simulink model "scenario1_TAC_5robots_plus_2019"  (R2019a)
settings: Solver=FixedStepAuto  StartTime=0.0  StopTime=40.0  FixedStep=1e-2  RelTol=1e-3
libraries: simulink x6
(part 2 of 2)

== matlab function scenario1_TAC_5robots_plus_2019/distance ==
  data: agent1_x1 input; distance_1_2 output; agent1_x2 input; agent2_x1 input; agent2_x2 input; agent3_x1 input; agent3_x2 input; agent4_x1 input; agent4_x2 input; agent5_x1 input; agent5_x2 input; distance_1_3 output; distance_1_4 output; distance_1_5 output; distance_2_3 output; distance_2_4 output; distance_2_5 output; distance_3_4 output; distance_3_5 output; distance_4_5 output
function [distance_1_2,distance_1_3,distance_1_4,distance_1_5,distance_2_3,distance_2_4,distance_2_5,distance_3_4,distance_3_5,distance_4_5]  = fcn(agent1_x1,agent1_x2,agent2_x1,agent2_x2,agent3_x1,agent3_x2,agent4_x1,agent4_x2,agent5_x1,agent5_x2)
distance_1_2=sqrt( (agent1_x1-agent2_x1)^2+ (agent1_x2-agent2_x2 )^2  );
distance_1_3=sqrt( (agent1_x1-agent3_x1)^2+ (agent1_x2-agent3_x2 )^2  );
distance_1_4=sqrt( (agent1_x1-agent4_x1)^2+ (agent1_x2-agent4_x2 )^2  );
distance_1_5=sqrt( (agent1_x1-agent5_x1)^2+ (agent1_x2-agent5_x2 )^2  );
distance_2_3=sqrt( (agent2_x1-agent3_x1)^2+ (agent2_x2-agent3_x2 )^2  );
distance_2_4=sqrt( (agent2_x1-agent4_x1)^2+ (agent2_x2-agent4_x2 )^2  );
distance_2_5=sqrt( (agent2_x1-agent5_x1)^2+ (agent2_x2-agent5_x2 )^2  );
distance_3_4=sqrt( (agent3_x1-agent4_x1)^2+ (agent3_x2-agent4_x2 )^2  );
distance_3_5=sqrt( (agent3_x1-agent5_x1)^2+ (agent3_x2-agent5_x2 )^2  );
distance_4_5=sqrt( (agent4_x1-agent5_x1)^2+ (agent4_x2-agent5_x2 )^2  );

== matlab function scenario1_TAC_5robots_plus_2019/agent_3/MATLAB Function ==
  data: x1 input; theta output; y1 input
function theta = fcn(x1, y1)
theta=atan2(y1,x1);

== matlab function scenario1_TAC_5robots_plus_2019/agent_3/MATLAB Function1 ==
  data: STL_u1 input; U1 output; STL_u2 input; STL_u3 input; PFM_u1 input; PFM_u2 input; PFM_u3 input; b1 input; U2 output; U3 output
function [U1,U2,U3] = fcn(STL_u1,STL_u2,STL_u3,PFM_u1,PFM_u2,PFM_u3,b1)
U_goal=[STL_u1;STL_u2;STL_u3];
U_obs=[PFM_u1;PFM_u2;PFM_u3];
k=0.15;
lambda=1-exp(-k*max(b1,0));
U=lambda*U_goal+(1-lambda)*U_obs;
U1=0;U2=0;U3=0;
U1=U(1,1);
U2=U(2,1);
U3=U(3,1);

== matlab function scenario1_TAC_5robots_plus_2019/agent_3/MATLAB Function2 ==
  data: v1 input; v output; v2 input
function v = fcn(v1, v2)
v=sqrt(v1^2+v2^2);

== matlab function scenario1_TAC_5robots_plus_2019/agent_3/Potential_Field_controller ==
  data: x1 input; x2 input; u1 output; xa3 input; agent1_x1 input; agent1_x2 input; agent2_x1 input; agent2_x2 input; agent4_x1 input; agent4_x2 input; agent5_x1 input; agent5_x2 input; t input; u2 output; u3 output; v_max input; yita output
function [u1,u2,u3,yita] = fcn(x1, x2, xa3,agent1_x1,agent1_x2,agent2_x1,agent2_x2,agent4_x1,agent4_x2,agent5_x1,agent5_x2,t,v_max)
coder.extrinsic('Calculate_gradient');
coder.extrinsic('Calculate_gradient_V1');
coder.extrinsic('Calculate_gradient_V1_yita');
coder.extrinsic('Calculate_gradient_static_d_1');
coder.extrinsic('Calculate_gradient_static_d_2');
coder.extrinsic('Calculate_gradient_dynamic');
coder.extrinsic('compute_convex_hull');
coder.extrinsic('PVF_optimizer');
coder.extrinsic('add_random');
yita=0;

A1=[-1,0;0,-1];
if t<20
    F=[100,0];
elseif t>=20 && t<41
     F=[200,200];
else
    F=[200,0];
end
obs=[50,50];
Robs_s=20;
r_obs=16;
distance=sqrt((x1-90)^2+(x2-90)^2);
gradient_x=0;gradient_y=0;
Dgradient_x=0;Dgradient_y=0;
agent1_gradient_x=0;agent1_gradient_y=0;
agent2_gradient_x=0;agent2_gradient_y=0;
agent4_gradient_x=0;agent4_gradient_y=0;
agent5_gradient_x=0;agent5_gradient_y=0;
[gradient_x,gradient_y]=Calculate_gradient(x1,x2,A1,F,50,50,Robs_s);
[agent1_gradient_x,agent1_gradient_y]=Calculate_gradient_dynamic(x1,x2,A1,F,agent1_x1,agent1_x2,10);
[agent2_gradient_x,agent2_gradient_y]=Calculate_gradient_dynamic(x1,x2,A1,F,agent2_x1,agent2_x2,10);
[agent4_gradient_x,agent4_gradient_y]=Calculate_gradient_dynamic(x1,x2,A1,F,agent4_x1,agent4_x2,10);
[agent5_gradient_x,agent5_gradient_y]=Calculate_gradient_dynamic(x1,x2,A1,F,agent5_x1,agent5_x2,10);
if sqrt((x1-agent1_x1)^2+(x2-agent1_x2)^2)<=30 %agent3 and agent1
     gradient_x=gradient_x+agent1_gradient_x;
     gradient_y=gradient_y+agent1_gradient_y;
end
if sqrt((x1-agent2_x1)^2+(x2-agent2_x2)^2)<=30 %agent3 and agent2
     gradient_x=gradient_x+agent2_gradient_x;
     gradient_y=gradient_y+agent2_gradient_y;
end
if sqrt((x1-agent4_x1)^2+(x2-agent4_x2)^2)<=30 %agent3 and agent4
     gradient_x=gradient_x+agent4_gradient_x;
     gradient_y=gradient_y+agent4_gradient_y;
end
if sqrt((x1-agent5_x1)^2+(x2-agent5_x2)^2)<=30 %agent3 and agent5
     gradient_x=gradient_x+agent5_gradient_x;
     gradient_y=gradient_y+agent5_gradient_y;
end
gradient_x=gradient_x;
gradient_y=gradient_y;  
gradient_z=0;
Gradient_all=[gradient_x;gradient_y;gradient_z];



Li=0.2;
Bi=[0,cos(pi/6),-cos(pi/6);
    -1,sin(pi/6),sin(pi/6);
    Li,Li,Li;];

R1=[cos(xa3),-sin(xa3),0;
    sin(xa3),cos(xa3),0;
    0,0,1;];
R=0.02;

gx=R1*inv(Bi')*R;
A=Gradient_all'*gx;
% A=[A;-gx];
%H=[1];
%H=[1,0;0,1];
%H=[0,0,0;0,0,0;0,0,0];

 H1=[1,0,0;0,1,0;0,0,0];
 H=(1/2)*gx'*H1*gx;
b=[0];
% b=[0;5000;5000;5000];
Gain=50;
Gradient_final=Gain*Gradient_all;
F=[-2*gx'*H1'*Gradient_final];
%=[];
u1=0;u2=0;u3=0;
U=PVF_optimizer(H,b,A,F,distance,gradient_x,gradient_y);

u1=U(1,1);
u2=U(2,1);
u3=U(3,1);

== matlab function scenario1_TAC_5robots_plus_2019/agent_3/STL_barrier  ==
  data: b output; b1 output; yita output; h output; t input; p1 input; p2 input; agent1_x1 input; agent1_x2 input; agent2_x1 input; agent2_x2 input; agent4_x1 input; agent4_x2 input; agent5_x1 input; agent5_x2 input
function [b,b1,yita,h] = fcn(t,p1,p2,agent1_x1,agent1_x2,agent2_x1,agent2_x2,agent4_x1,agent4_x2,agent5_x1,agent5_x2)
if t<20
    d1=50;
    d2=0;
elseif t>=20 && t<41
    d1=100;
    d2=100;
else
    d1=100;
    d2=0;  
end

obs1=50;
obs2=50;
if t<20
b=105*exp(-0.22*t)+5-sqrt( (p1-d1)^2 + (p2-d2)^2 );
yita=-105*exp(-0.22*t)+5;
h=10-sqrt( (p1-d1)^2 + (p2-d2)^2 );
elseif t>=20 && t<41
    b=110*exp(-0.22*(t-20))+5-sqrt( (p1-d1)^2 + (p2-d2)^2 );
   yita=-110*exp(-0.22*(t-20))+5;
    h=10-sqrt( (p1-d1)^2 + (p2-d2)^2 );
else
   b=145*exp(-0.24*(t-40))+5-sqrt( (p1-d1)^2 + (p2-d2)^2 );
   yita=-145*exp(-0.24*(t-40))+5;
   h=10-sqrt( (p1-d1)^2 + (p2-d2)^2 );
end
% b11=sqrt( (p1-x1_agent2)^2 + (p2-x2_agent2)^2 )-10 %collision avoidence with agent2
bobs=sqrt( (p1-obs1)^2 + (p2-obs2)^2 )-20;%collision avoidence with obstacle (50,50)
b31=sqrt( (p1-agent1_x1)^2 + (p2-agent1_x2)^2 )-10;%collision avoidence with agent1
b32=sqrt( (p1-agent2_x1)^2 + (p2-agent2_x2)^2 )-10;%collision avoidence with agent2
b34=sqrt( (p1-agent4_x1)^2 + (p2-agent4_x2)^2 )-10;%collision avoidence with agent4
b35=sqrt( (p1-agent5_x1)^2 + (p2-agent5_x2)^2 )-10;%collision avoidence with agent5
% b13=sqrt( (p1-centerjk_1)^2 + (p2-centerjk_2)^2 )-R_jk_s;%collision avoidence with nominal
% b14=sqrt( (p1-60)^2 + (p2-85)^2 )-18; %static dynamic obstacle
% b15=sqrt( (p1-20)^2 + (p2-80)^2 )-10; %static dynamic obstacle


b1=-(1/20)*log(exp(-20*bobs)+exp(-20*b31)+exp(-20*b32)+exp(-20*b34)+exp(-20*b35));

% b1=-(1/20)*log(exp(-20*b11)+exp(-20*b12)+exp(-20*b14)+exp(-20*b15));%+log(2);

== matlab function scenario1_TAC_5robots_plus_2019/agent_3/STL_controller ==
  data: x1 input; x2 input; b_in input; u1 output; xa3 input; u2 output; u3 output; t input; v_max input
function [u1,u2,u3]= fcn(x1, x2, b_in, xa3,t, v_max)
coder.extrinsic('quadoptimizer');
%coder.extrinsic('save');
if t<20
    d1=50; d2=0;
elseif t>=20 && t<41
   d1=100; d2=100; 
else
   d1=100; d2=0; 
end

partial_b=(1/2)*((x1-d1)^2+(x2-d2)^2)^(-1/2);
partial_b_x=[-2*partial_b*(x1-d1),-2*partial_b*(x2-d2),0];


Li=0.2;
Bi=[0,cos(pi/6),-cos(pi/6);
    -1,sin(pi/6),sin(pi/6);
    Li,Li,Li;];

R1=[cos(xa3),-sin(xa3),0;
    sin(xa3),cos(xa3),0;
    0,0,1;];
R=0.02;
gx=R1*inv(Bi')*R;

A=partial_b_x*gx;
% A=[A;-gx];
H=[1,0,0;0,1,0;0,0,1];
%H=[1];
if t<20
    b=5*b_in-0.22*105*exp(-0.22*t)-20;
elseif t>=20 && t<41
    b=5*b_in-0.22*110*exp(-0.22*(t-20))-20;
else
    b=20*b_in-0.24*145*exp(-0.24*(t-40))-100;
end
% b=[b;5000;5000;5000];


u1=0;u2=0;u3=0;
U=[0;0;0];
U=quadoptimizer(H,b,A);

%U=quadprod(H,[],-A,b);
% V=[0;0;0];
% V=gx*U;
% if V(1,1)^2+V(2,1)^2<=v_max^2
%      U(1,1)= U(1,1);
%      U(2,1)= U(2,1);
% else 
%     U(1,1)=sqrt(v_max^2/(V(1,1)^2+V(2,1)^2))*U(1,1);
%     U(2,1)=sqrt(v_max^2/(V(1,1)^2+V(2,1)^2))*U(2,1);
% end


u1=U(1,1);
u2=U(2,1);
u3=U(3,1);

== matlab function scenario1_TAC_5robots_plus_2019/agent_3/omnidirectional robot_1 ==
  data: ua1 input; xa1_dot output; ua2 input; ua3 input; xa3 input; xa2_dot output; xa3_dot output
function [xa1_dot,xa2_dot,xa3_dot]= fcn(ua1,ua2,ua3,xa3)

Li=0.2;
Bi=[0,cos(pi/6),-cos(pi/6);
    -1,sin(pi/6),sin(pi/6);
    Li,Li,Li;];

R1=[cos(xa3),-sin(xa3),0;
    sin(xa3),cos(xa3),0;
    0,0,1;];
R=0.02;
A=R1*inv(Bi')*R*[ua1;ua2;ua3];
xa1_dot=A(1,1);
xa2_dot=A(2,1);
xa3_dot=A(3,1);

== matlab function scenario1_TAC_5robots_plus_2019/agent_3/velocity_constraint ==
  data: U1 input; Uc1 output; U2 input; U3 input; Uc2 output; Uc3 output; xa3 input; v_max input
function [Uc1,Uc2,Uc3] = fcn(U1,U2,U3,xa3,v_max)

Li=0.2;
Bi=[0,cos(pi/6),-cos(pi/6);
    -1,sin(pi/6),sin(pi/6);
    Li,Li,Li;];

R1=[cos(xa3),-sin(xa3),0;
    sin(xa3),cos(xa3),0;
    0,0,1;];
R=0.02;
gx=R1*inv(Bi')*R;

U=[U1;U2;U3];
V=[0;0;0];
V=gx*U;
if V(1,1)^2+V(2,1)^2<=v_max^2
     U(1,1)= U(1,1);
     U(2,1)= U(2,1);
else 
    U(1,1)=sqrt(v_max^2/(V(1,1)^2+V(2,1)^2))*U(1,1);
    U(2,1)=sqrt(v_max^2/(V(1,1)^2+V(2,1)^2))*U(2,1);
    U(3,1)=sqrt(v_max^2/(V(1,1)^2+V(2,1)^2))*U(3,1);
end

Uc1=U(1,1);
Uc2=U(2,1);
Uc3=U(3,1);

== matlab function scenario1_TAC_5robots_plus_2019/agent_4/MATLAB Function ==
  data: x1 input; theta output; y1 input
function theta = fcn(x1, y1)
theta=atan2(y1,x1);

== matlab function scenario1_TAC_5robots_plus_2019/agent_4/MATLAB Function1 ==
  data: STL_u1 input; U1 output; STL_u2 input; STL_u3 input; PFM_u1 input; PFM_u2 input; PFM_u3 input; b1 input; U2 output; U3 output; t input
function [U1,U2,U3] = fcn(STL_u1,STL_u2,STL_u3,PFM_u1,PFM_u2,PFM_u3,b1,t)
U_goal=[STL_u1;STL_u2;STL_u3];
U_obs=[PFM_u1;PFM_u2;PFM_u3];
k=0.15;
lambda=1-exp(-k*max(b1,0));
U=lambda*U_goal+(1-lambda)*U_obs;
U1=0;U2=0;U3=0;
if t<=20
U1=0;
U2=0;
U3=0;    
% U1=U(1,1);
% U2=U(2,1);
% U3=U(3,1);
else
U1=U(1,1);
U2=U(2,1);
U3=U(3,1);
end

== matlab function scenario1_TAC_5robots_plus_2019/agent_4/MATLAB Function2 ==
  data: v1 input; v output; v2 input
function v = fcn(v1, v2)
v=sqrt(v1^2+v2^2);

== matlab function scenario1_TAC_5robots_plus_2019/agent_4/Potential_Field_controller ==
  data: x1 input; x2 input; u1 output; xa3 input; agent1_x1 input; agent1_x2 input; agent2_x1 input; agent2_x2 input; agent3_x1 input; agent3_x2 input; agent5_x1 input; agent5_x2 input; t input; u2 output; u3 output; v_max input; yita output
function [u1,u2,u3,yita] = fcn(x1, x2, xa3,agent1_x1,agent1_x2,agent2_x1,agent2_x2,agent3_x1,agent3_x2,agent5_x1,agent5_x2,t,v_max)
coder.extrinsic('Calculate_gradient');
coder.extrinsic('Calculate_gradient_V1');
coder.extrinsic('Calculate_gradient_V1_yita');
coder.extrinsic('Calculate_gradient_static_d_1');
coder.extrinsic('Calculate_gradient_static_d_2');
coder.extrinsic('Calculate_gradient_dynamic');
coder.extrinsic('compute_convex_hull');
coder.extrinsic('PVF_optimizer');
coder.extrinsic('add_random');
yita=0;

A1=[-1,0;0,-1];
if t<20
    F=[2*(-45*cos(t)+50),2*(45*sin(t)+50)];
elseif t>=20 && t<41
%      F=[0,200];
    F=[2*(-45*cos(t-20)+50),2*(45*sin(t-20)+50)];
else
    F=[200,0];
end
obs=[50,50];
Robs_s=20;
r_obs=16;
distance=sqrt((x1-90)^2+(x2-90)^2);
gradient_x=0;gradient_y=0;
Dgradient_x=0;Dgradient_y=0;
agent1_gradient_x=0;agent1_gradient_y=0;
agent2_gradient_x=0;agent2_gradient_y=0;
agent3_gradient_x=0;agent3_gradient_y=0;
agent5_gradient_x=0;agent5_gradient_y=0;
[gradient_x,gradient_y]=Calculate_gradient(x1,x2,A1,F,50,50,Robs_s);
[agent1_gradient_x,agent1_gradient_y]=Calculate_gradient_dynamic(x1,x2,A1,F,agent1_x1,agent1_x2,10);
[agent2_gradient_x,agent2_gradient_y]=Calculate_gradient_dynamic(x1,x2,A1,F,agent2_x1,agent2_x2,10);
[agent3_gradient_x,agent3_gradient_y]=Calculate_gradient_dynamic(x1,x2,A1,F,agent3_x1,agent3_x2,10);
[agent5_gradient_x,agent5_gradient_y]=Calculate_gradient_dynamic(x1,x2,A1,F,agent5_x1,agent5_x2,10);
if sqrt((x1-agent1_x1)^2+(x2-agent1_x2)^2)<=30 %agent4 and agent1
     gradient_x=gradient_x+agent1_gradient_x;
     gradient_y=gradient_y+agent1_gradient_y;
end
if sqrt((x1-agent2_x1)^2+(x2-agent2_x2)^2)<=30 %agent4 and agent2
     gradient_x=gradient_x+agent2_gradient_x;
     gradient_y=gradient_y+agent2_gradient_y;
end
if sqrt((x1-agent3_x1)^2+(x2-agent3_x2)^2)<=30 %agent4 and agent3
     gradient_x=gradient_x+agent3_gradient_x;
     gradient_y=gradient_y+agent3_gradient_y;
end
if sqrt((x1-agent5_x1)^2+(x2-agent5_x2)^2)<=30 %agent4 and agent5
     gradient_x=gradient_x+agent5_gradient_x;
     gradient_y=gradient_y+agent5_gradient_y;
end
gradient_x=gradient_x;
gradient_y=gradient_y;  
gradient_z=0;
Gradient_all=[gradient_x;gradient_y;gradient_z];



Li=0.2;
Bi=[0,cos(pi/6),-cos(pi/6);
    -1,sin(pi/6),sin(pi/6);
    Li,Li,Li;];

R1=[cos(xa3),-sin(xa3),0;
    sin(xa3),cos(xa3),0;
    0,0,1;];
R=0.02;

gx=R1*inv(Bi')*R;
A=Gradient_all'*gx;
% A=[A;-gx];
%H=[1];
%H=[1,0;0,1];
%H=[0,0,0;0,0,0;0,0,0];

 H1=[1,0,0;0,1,0;0,0,0];
 H=(1/2)*gx'*H1*gx;
b=[0];
% b=[0;5000;5000;5000];
Gain=50;
Gradient_final=Gain*Gradient_all;
F=[-2*gx'*H1'*Gradient_final];
%=[];
u1=0;u2=0;u3=0;
U=PVF_optimizer(H,b,A,F,distance,gradient_x,gradient_y);

u1=U(1,1);
u2=U(2,1);
u3=U(3,1);

== matlab function scenario1_TAC_5robots_plus_2019/agent_4/STL_barrier  ==
  data: b output; b1 output; yita output; h output; t input; p1 input; p2 input; agent1_x1 input; agent1_x2 input; agent2_x1 input; agent2_x2 input; agent3_x1 input; agent3_x2 input; agent5_x1 input; agent5_x2 input
function [b,b1,yita,h] = fcn(t,p1,p2,agent1_x1,agent1_x2,agent2_x1,agent2_x2,agent3_x1,agent3_x2,agent5_x1,agent5_x2)
if t<20
    d1=-45*cos(t)+50;
    d2= 45*sin(t)+50;
elseif t>=20 && t<41
    d1=-45*cos(t-20)+50;
    d2= 45*sin(t-20)+50;
else
    d1=100;
    d2=0;  
end

obs1=50;
obs2=50;
if t<20
% b=105*exp(-0.22*t)+5-sqrt( (p1-d1)^2 + (p2-d2)^2 );
% yita=-105*exp(-0.22*t)+5;
% h=10-sqrt( (p1-d1)^2 + (p2-d2)^2 );
b=7-sqrt( (p1-d1)^2 + (p2-d2)^2 );
yita=3;
h=10-sqrt( (p1-d1)^2 + (p2-d2)^2 );
elseif t>=20 && t<41
%     b=90*exp(-0.208*(t-20))+5-sqrt( (p1-d1)^2 + (p2-d2)^2 );
%    yita=-90*exp(-0.2295*(t-20))+5;
%     h=10-sqrt( (p1-d1)^2 + (p2-d2)^2 );
b=7-sqrt( (p1-d1)^2 + (p2-d2)^2 );
yita=3;
h=10-sqrt( (p1-d1)^2 + (p2-d2)^2 );
else
   b=145*exp(-0.24*(t-40))+5-sqrt( (p1-d1)^2 + (p2-d2)^2 );
   yita=-145*exp(-0.24*(t-40))+5;
   h=10-sqrt( (p1-d1)^2 + (p2-d2)^2 );
end
bobs=sqrt( (p1-obs1)^2 + (p2-obs2)^2 )-20;%collision avoidence with obstacle (50,50)
b41=sqrt( (p1-agent1_x1)^2 + (p2-agent1_x2)^2 )-10;%collision avoidence with agent1
b42=sqrt( (p1-agent2_x1)^2 + (p2-agent2_x2)^2 )-10;%collision avoidence with agent2
b43=sqrt( (p1-agent3_x1)^2 + (p2-agent3_x2)^2 )-10;%collision avoidence with agent3
b45=sqrt( (p1-agent5_x1)^2 + (p2-agent5_x2)^2 )-10;%collision avoidence with agent5

b1=-(1/20)*log(exp(-20*bobs)+exp(-20*b41)+exp(-20*b42)+exp(-20*b43)+exp(-20*b45));

% b1=-(1/20)*log(exp(-20*b11)+exp(-20*b12)+exp(-20*b14)+exp(-20*b15));%+log(2);

== matlab function scenario1_TAC_5robots_plus_2019/agent_4/STL_controller ==
  data: x1 input; x2 input; b_in input; u1 output; xa3 input; u2 output; u3 output; t input; v_max input
function [u1,u2,u3]= fcn(x1, x2, b_in, xa3,t, v_max)
coder.extrinsic('quadoptimizer');
%coder.extrinsic('save');
if t<20
    d1=-45*cos(t)+50; d2=45*sin(t)+50;
elseif t>=20 && t<41
%    d1=0; d2=100; 
    d1=-45*cos(t-20)+50; d2=45*sin(t-20)+50;
else
   d1=100; d2=0; 
end

partial_b=(1/2)*((x1-d1)^2+(x2-d2)^2)^(-1/2);
partial_b_x=[-2*partial_b*(x1-d1),-2*partial_b*(x2-d2),0];
partial_b_t= -2*partial_b*(x1-d1)*(-45*sin(t-20))-2*partial_b*(x2-d2)*(-45*cos(t-20));

Li=0.2;
Bi=[0,cos(pi/6),-cos(pi/6);
    -1,sin(pi/6),sin(pi/6);
    Li,Li,Li;];

R1=[cos(xa3),-sin(xa3),0;
    sin(xa3),cos(xa3),0;
    0,0,1;];
R=0.02;
gx=R1*inv(Bi')*R;

A=partial_b_x*gx;
% A=[A;-gx];
H=[1,0,0;0,1,0;0,0,1];
%H=[1];
if t<20
%     b=5*b_in-0.22*105*exp(-0.22*t)-20;
     b=5*b_in+partial_b_t-10;
elseif t>=20 && t<41
%     b=20*b_in-0.208*90*exp(-0.208*(t-20))-100;
     b=50*b_in+partial_b_t-50;
else
    b=20*b_in-0.24*145*exp(-0.24*(t-40))-100;
end
% b=[b;5000;5000;5000];


u1=0;u2=0;u3=0;
U=[0;0;0];
U=quadoptimizer(H,b,A);

%U=quadprod(H,[],-A,b);
% V=[0;0;0];
% V=gx*U;
% if V(1,1)^2+V(2,1)^2<=v_max^2
%      U(1,1)= U(1,1);
%      U(2,1)= U(2,1);
% else 
%     U(1,1)=sqrt(v_max^2/(V(1,1)^2+V(2,1)^2))*U(1,1);
%     U(2,1)=sqrt(v_max^2/(V(1,1)^2+V(2,1)^2))*U(2,1);
% end


u1=U(1,1);
u2=U(2,1);
u3=U(3,1);

== matlab function scenario1_TAC_5robots_plus_2019/agent_4/omnidirectional robot_1 ==
  data: ua1 input; xa1_dot output; ua2 input; ua3 input; xa3 input; xa2_dot output; xa3_dot output
function [xa1_dot,xa2_dot,xa3_dot]= fcn(ua1,ua2,ua3,xa3)

Li=0.2;
Bi=[0,cos(pi/6),-cos(pi/6);
    -1,sin(pi/6),sin(pi/6);
    Li,Li,Li;];

R1=[cos(xa3),-sin(xa3),0;
    sin(xa3),cos(xa3),0;
    0,0,1;];
R=0.02;
A=R1*inv(Bi')*R*[ua1;ua2;ua3];
xa1_dot=A(1,1);
xa2_dot=A(2,1);
xa3_dot=A(3,1);

== matlab function scenario1_TAC_5robots_plus_2019/agent_4/velocity_constraint ==
  data: U1 input; Uc1 output; U2 input; U3 input; Uc2 output; Uc3 output; xa3 input; v_max input
function [Uc1,Uc2,Uc3] = fcn(U1,U2,U3,xa3,v_max)

Li=0.2;
Bi=[0,cos(pi/6),-cos(pi/6);
    -1,sin(pi/6),sin(pi/6);
    Li,Li,Li;];

R1=[cos(xa3),-sin(xa3),0;
    sin(xa3),cos(xa3),0;
    0,0,1;];
R=0.02;
gx=R1*inv(Bi')*R;

U=[U1;U2;U3];
V=[0;0;0];
V=gx*U;
if V(1,1)^2+V(2,1)^2<=v_max^2
     U(1,1)= U(1,1);
     U(2,1)= U(2,1);
else 
    U(1,1)=sqrt(v_max^2/(V(1,1)^2+V(2,1)^2))*U(1,1);
    U(2,1)=sqrt(v_max^2/(V(1,1)^2+V(2,1)^2))*U(2,1);
    U(3,1)=sqrt(v_max^2/(V(1,1)^2+V(2,1)^2))*U(3,1);
end

Uc1=U(1,1);
Uc2=U(2,1);
Uc3=U(3,1);

== matlab function scenario1_TAC_5robots_plus_2019/agent_5/MATLAB Function ==
  data: x1 input; theta output; y1 input
function theta = fcn(x1, y1)
theta=atan2(y1,x1);

== matlab function scenario1_TAC_5robots_plus_2019/agent_5/MATLAB Function1 ==
  data: STL_u1 input; U1 output; STL_u2 input; STL_u3 input; PFM_u1 input; PFM_u2 input; PFM_u3 input; b1 input; U2 output; U3 output
function [U1,U2,U3] = fcn(STL_u1,STL_u2,STL_u3,PFM_u1,PFM_u2,PFM_u3,b1)
U_goal=[STL_u1;STL_u2;STL_u3];
U_obs=[PFM_u1;PFM_u2;PFM_u3];
k=0.15;
lambda=1-exp(-k*max(b1,0));
U=lambda*U_goal+(1-lambda)*U_obs;
U1=0;U2=0;U3=0;
U1=U(1,1);
U2=U(2,1);
U3=U(3,1);

== matlab function scenario1_TAC_5robots_plus_2019/agent_5/MATLAB Function2 ==
  data: v1 input; v output; v2 input
function v = fcn(v1, v2)
v=sqrt(v1^2+v2^2);

== matlab function scenario1_TAC_5robots_plus_2019/agent_5/Potential_Field_controller ==
  data: x1 input; x2 input; u1 output; xa3 input; agent1_x1 input; agent1_x2 input; agent2_x1 input; agent2_x2 input; agent3_x1 input; agent3_x2 input; agent4_x1 input; agent4_x2 input; t input; u2 output; u3 output; v_max input; yita output
function [u1,u2,u3,yita] = fcn(x1, x2, xa3,agent1_x1,agent1_x2,agent2_x1,agent2_x2,agent3_x1,agent3_x2,agent4_x1,agent4_x2,t,v_max)
coder.extrinsic('Calculate_gradient');
coder.extrinsic('Calculate_gradient_V1');
coder.extrinsic('Calculate_gradient_V1_yita');
coder.extrinsic('Calculate_gradient_static_d_1');
coder.extrinsic('Calculate_gradient_static_d_2');
coder.extrinsic('Calculate_gradient_dynamic');
coder.extrinsic('compute_convex_hull');
coder.extrinsic('PVF_optimizer');
coder.extrinsic('add_random');
yita=0;

A1=[-1,0;0,-1];
if t<20
    F=[200,0];
elseif t>=20 && t<41
     F=[210,200];
else
    F=[200,0];
end
obs=[50,50];
Robs_s=20;
r_obs=16;
distance=sqrt((x1-90)^2+(x2-90)^2);
gradient_x=0;gradient_y=0;
Dgradient_x=0;Dgradient_y=0;
agent1_gradient_x=0;agent1_gradient_y=0;
agent2_gradient_x=0;agent2_gradient_y=0;
[gradient_x,gradient_y]=Calculate_gradient(x1,x2,A1,F,50,50,Robs_s);
[agent1_gradient_x,agent1_gradient_y]=Calculate_gradient_dynamic(x1,x2,A1,F,agent1_x1,agent1_x2,10);
[agent2_gradient_x,agent2_gradient_y]=Calculate_gradient_dynamic(x1,x2,A1,F,agent2_x1,agent2_x2,10);
if sqrt((x1-agent1_x1)^2+(x2-agent1_x2)^2)<=30 %agent3 and agent1
     gradient_x=gradient_x+agent1_gradient_x;
     gradient_y=gradient_y+agent1_gradient_y;
end
if sqrt((x1-agent2_x1)^2+(x2-agent2_x2)^2)<=30 %agent3 and agent2
     gradient_x=gradient_x+agent2_gradient_x;
     gradient_y=gradient_y+agent2_gradient_y;
end
gradient_x=gradient_x;
gradient_y=gradient_y;  
gradient_z=0;
Gradient_all=[gradient_x;gradient_y;gradient_z];



Li=0.2;
Bi=[0,cos(pi/6),-cos(pi/6);
    -1,sin(pi/6),sin(pi/6);
    Li,Li,Li;];

R1=[cos(xa3),-sin(xa3),0;
    sin(xa3),cos(xa3),0;
    0,0,1;];
R=0.02;

gx=R1*inv(Bi')*R;
A=Gradient_all'*gx;
% A=[A;-gx];
%H=[1];
%H=[1,0;0,1];
%H=[0,0,0;0,0,0;0,0,0];

 H1=[1,0,0;0,1,0;0,0,0];
 H=(1/2)*gx'*H1*gx;
b=[0];
% b=[0;5000;5000;5000];
Gain=50;
Gradient_final=Gain*Gradient_all;
F=[-2*gx'*H1'*Gradient_final];
%=[];
u1=0;u2=0;u3=0;
U=PVF_optimizer(H,b,A,F,distance,gradient_x,gradient_y);

u1=U(1,1);
u2=U(2,1);
u3=U(3,1);

== matlab function scenario1_TAC_5robots_plus_2019/agent_5/STL_barrier  ==
  data: b output; b1 output; yita output; h output; t input; p1 input; p2 input; agent1_x1 input; agent1_x2 input; agent2_x1 input; agent2_x2 input; agent3_x1 input; agent3_x2 input; agent4_x1 input; agent4_x2 input; yita_1 output; h_1 output
function [b,b1,yita,h,yita_1,h_1] = fcn(t,p1,p2,agent1_x1,agent1_x2,agent2_x1,agent2_x2,agent3_x1,agent3_x2,agent4_x1,agent4_x2)
d11=0;d22=0;
if t<20
    d1=100;
    d2=0;
elseif t>=20 && t<41
    d1=100;d2=100;
    d11=110;d22=100;
else
    d1=100;
    d2=0;  
end
yita_1=0;h_1=0;
obs1=50;
obs2=50;
if t<20
b=145*exp(-0.24*t)+5-sqrt( (p1-d1)^2 + (p2-d2)^2 );
yita=-145*exp(-0.24*t)+5;
h=10-sqrt( (p1-d1)^2 + (p2-d2)^2 );
elseif t>=20 && t<41
   b_1=100*exp(-0.215*(t-20))+5-sqrt( (p1-d1)^2 + (p2-d2)^2 );
   yita_1=-100*exp(-0.215*(t-20))+5;
   h_1=10-sqrt( (p1-d1)^2 + (p2-d2)^2 );
   
   b_2=100*exp(-0.215*(t-20))+5-sqrt( (p1-d11)^2 + (p2-d22)^2 );
   yita=-100*exp(-0.215*(t-20))+5;
   h=10-sqrt( (p1-d11)^2 + (p2-d22)^2 );
   b=-(1/20)*log(exp(-20*b_1)+exp(-20*b_2));
else
   b=145*exp(-0.24*(t-40))+5-sqrt( (p1-d1)^2 + (p2-d2)^2 );
   yita=-145*exp(-0.24*(t-40))+5;
   h=10-sqrt( (p1-d1)^2 + (p2-d2)^2 );
end
bobs=sqrt( (p1-obs1)^2 + (p2-obs2)^2 )-20;%collision avoidence with obstacle (50,50)
b51=sqrt( (p1-agent1_x1)^2 + (p2-agent1_x2)^2 )-10;%collision avoidence with agent1
b52=sqrt( (p1-agent2_x1)^2 + (p2-agent2_x2)^2 )-10;%collision avoidence with agent2
b53=sqrt( (p1-agent3_x1)^2 + (p2-agent3_x2)^2 )-10;%collision avoidence with agent3
b54=sqrt( (p1-agent4_x1)^2 + (p2-agent4_x2)^2 )-10;%collision avoidence with agent4


b1=-(1/20)*log(exp(-20*bobs)+exp(-20*b51)+exp(-20*b52)+exp(-20*b53)+exp(-20*b54));

% b1=-(1/20)*log(exp(-20*b11)+exp(-20*b12)+exp(-20*b14)+exp(-20*b15));%+log(2);

== matlab function scenario1_TAC_5robots_plus_2019/agent_5/STL_controller ==
  data: x1 input; x2 input; b_in input; u1 output; xa3 input; u2 output; u3 output; t input; v_max input
function [u1,u2,u3]= fcn(x1, x2, b_in, xa3,t, v_max)
coder.extrinsic('quadoptimizer');
%coder.extrinsic('save');
d11=0;d22=0;
b_1=0;b_2=0;partial_b_t=0;
if t<20
    d1=100; d2=0;
elseif t>=20 && t<41
   d1=100; d2=100; 
   d11=110;d22=100;
   b_1=100*exp(-0.215*(t-20))+5-sqrt( (x1-d1)^2 + (x2-d2)^2 );
   b_2=100*exp(-0.215*(t-20))+5-sqrt( (x1-d11)^2 + (x2-d22)^2 );
else
   d1=100; d2=0; 
end

if t<20
partial_b=(1/2)*((x1-d1)^2+(x2-d2)^2)^(-1/2);
partial_b_x=[-2*partial_b*(x1-d1),-2*partial_b*(x2-d2),0];
else
partial_b1=(1/2)*((x1-d1)^2+(x2-d2)^2)^(-1/2);
partial_b1_x=[-2*partial_b1*(x1-d1),-2*partial_b1*(x2-d2),0];

partial_b2=(1/2)*((x1-d11)^2+(x2-d22)^2)^(-1/2);
partial_b2_x=[-2*partial_b2*(x1-d11),-2*partial_b2*(x2-d22),0];

partial_b_b1=exp(-20*b_1)/( exp(-20*b_1) + exp(-20*b_2) );
partial_b_b2=exp(-20*b_2)/( exp(-20*b_1) + exp(-20*b_2) );
partial_b_x= partial_b_b1* partial_b1_x + partial_b_b2*partial_b2_x;
partial_b_t= partial_b_b1*(-0.215*100*exp(-0.215*(t-20))) + partial_b_b2*(-0.215*100*exp(-0.215*(t-20)));
end


Li=0.2;
Bi=[0,cos(pi/6),-cos(pi/6);
    -1,sin(pi/6),sin(pi/6);
    Li,Li,Li;];

R1=[cos(xa3),-sin(xa3),0;
    sin(xa3),cos(xa3),0;
    0,0,1;];
R=0.02;
gx=R1*inv(Bi')*R;

A=partial_b_x*gx;
% A=[A;-gx];
H=[1,0,0;0,1,0;0,0,1];
%H=[1];
if t<20
    b=5*b_in-0.24*145*exp(-0.24*t)-20;
elseif t>=20 && t<41
    b=5*b_in + partial_b_t - 20;
else
    b=20*b_in-0.24*145*exp(-0.24*(t-40))-100;
end
% b=[b;5000;5000;5000];


u1=0;u2=0;u3=0;
U=[0;0;0];
U=quadoptimizer(H,b,A);

%U=quadprod(H,[],-A,b);
% V=[0;0;0];
% V=gx*U;
% if V(1,1)^2+V(2,1)^2<=v_max^2
%      U(1,1)= U(1,1);
%      U(2,1)= U(2,1);
% else 
%     U(1,1)=sqrt(v_max^2/(V(1,1)^2+V(2,1)^2))*U(1,1);
%     U(2,1)=sqrt(v_max^2/(V(1,1)^2+V(2,1)^2))*U(2,1);
% end


u1=U(1,1);
u2=U(2,1);
u3=U(3,1);

== matlab function scenario1_TAC_5robots_plus_2019/agent_5/omnidirectional robot_1 ==
  data: ua1 input; xa1_dot output; ua2 input; ua3 input; xa3 input; xa2_dot output; xa3_dot output
function [xa1_dot,xa2_dot,xa3_dot]= fcn(ua1,ua2,ua3,xa3)

Li=0.2;
Bi=[0,cos(pi/6),-cos(pi/6);
    -1,sin(pi/6),sin(pi/6);
    Li,Li,Li;];

R1=[cos(xa3),-sin(xa3),0;
    sin(xa3),cos(xa3),0;
    0,0,1;];
R=0.02;
A=R1*inv(Bi')*R*[ua1;ua2;ua3];
xa1_dot=A(1,1);
xa2_dot=A(2,1);
xa3_dot=A(3,1);

== matlab function scenario1_TAC_5robots_plus_2019/agent_5/velocity_constraint ==
  data: U1 input; Uc1 output; U2 input; U3 input; Uc2 output; Uc3 output; xa3 input; v_max input
function [Uc1,Uc2,Uc3] = fcn(U1,U2,U3,xa3,v_max)

Li=0.2;
Bi=[0,cos(pi/6),-cos(pi/6);
    -1,sin(pi/6),sin(pi/6);
    Li,Li,Li;];

R1=[cos(xa3),-sin(xa3),0;
    sin(xa3),cos(xa3),0;
    0,0,1;];
R=0.02;
gx=R1*inv(Bi')*R;

U=[U1;U2;U3];
V=[0;0;0];
V=gx*U;
if V(1,1)^2+V(2,1)^2<=v_max^2
     U(1,1)= U(1,1);
     U(2,1)= U(2,1);
else 
    U(1,1)=sqrt(v_max^2/(V(1,1)^2+V(2,1)^2))*U(1,1);
    U(2,1)=sqrt(v_max^2/(V(1,1)^2+V(2,1)^2))*U(2,1);
    U(3,1)=sqrt(v_max^2/(V(1,1)^2+V(2,1)^2))*U(3,1);
end

Uc1=U(1,1);
Uc2=U(2,1);
Uc3=U(3,1);

== matlab function scenario1_TAC_5robots_plus_2019/agent_4/MATLAB Function3 ==
  data: t input; L1 output; L2 output
function [L1,L2] = fcn(t)
if t<20
    L1=0;
    L2=50;
else
    L1=-45*cos(t-20)+50;
    L2= 45*sin(t-20)+50;
end
